simulink model "mg327337"  (Simulink 6.5)
settings: Solver=FixedStepDiscrete  StartTime=0.0  StopTime=20  FixedStep=1  RelTol=1e-3
libraries: simulink x6
CloseFcn:
  | rtwprivate ssgensfun ModelCloseRequest mg327337
settings Model: Creator=mshakeri  LastModifiedBy=mshakeri  ExtModeAutoUpdateStatusClock=off
settings OptimizationCC: InlineParams=on
settings DebuggingCC: SignalResolutionControl=UseLocalSettings  StrictBusMsg=ErrorLevel1

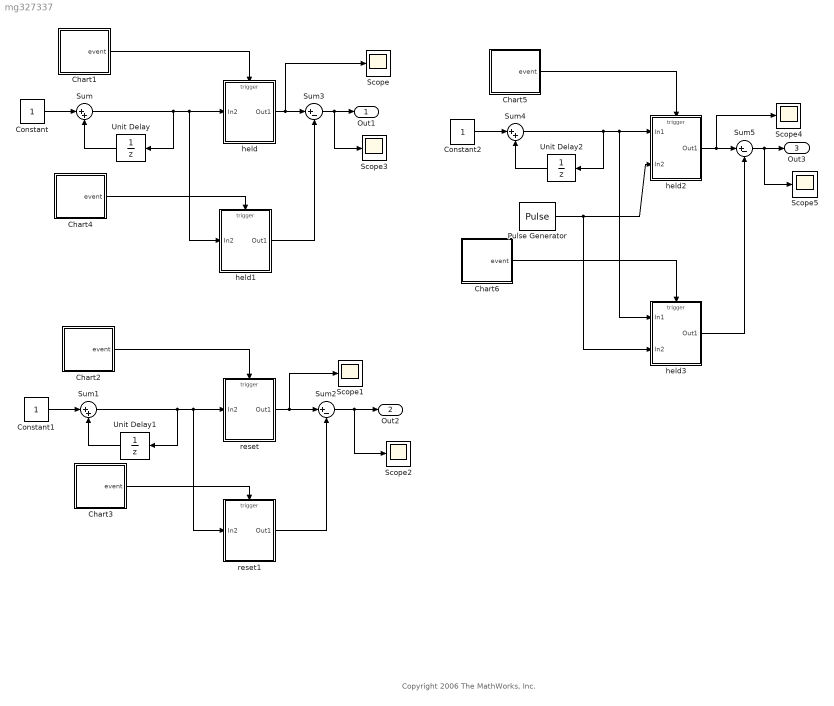
== system mg327337 ==
  note: Copyright 2006 The MathWorks, Inc.
  Chart1 : Stateflow chart  TreatAsAtomicUnit=on  SystemSampleTime=1
  Chart2 : Stateflow chart  TreatAsAtomicUnit=on  SystemSampleTime=1
  Chart3 : Stateflow chart  TreatAsAtomicUnit=on  SystemSampleTime=1
  Chart4 : Stateflow chart  TreatAsAtomicUnit=on  SystemSampleTime=1
  Chart5 : Stateflow chart  TreatAsAtomicUnit=on  SystemSampleTime=1
  Chart6 : Stateflow chart  TreatAsAtomicUnit=on  SystemSampleTime=1
  Constant : Constant
  Constant1 : Constant
  Constant2 : Constant
  Pulse Generator : DiscretePulseGenerator  PulseType=Time based  PulseWidth=50
  Scope{,1..5} (6 alike) : Scope
      Scope2 settings: SaveName=ScopeData2
      Scope3 settings: SaveName=ScopeData3
      Scope4 settings: SaveName=ScopeData4
      Scope5 settings: SaveName=ScopeData5
  Sum : Sum  Inputs=|++
  Sum1 : Sum  Inputs=|++
  Sum2 : Sum  Inputs=|+-
  Sum3 : Sum  Inputs=|+-
  Sum4 : Sum  Inputs=|++
  Sum5 : Sum  Inputs=|+-
  Unit Delay : UnitDelay  Orientation=left
  Unit Delay1 : UnitDelay  Orientation=left
  Unit Delay2 : UnitDelay  Orientation=left
  held : Subsystem  TreatAsAtomicUnit=on
      settings: RTWSystemCode=Inline
  held1 : Subsystem  TreatAsAtomicUnit=on
      settings: RTWSystemCode=Inline
  held2 : Subsystem  TreatAsAtomicUnit=on
      settings: RTWSystemCode=Inline
  held3 : Subsystem  TreatAsAtomicUnit=on
      settings: RTWSystemCode=Inline
  reset : Subsystem  TreatAsAtomicUnit=on
      settings: RTWSystemCode=Inline
  reset1 : Subsystem  TreatAsAtomicUnit=on
      settings: RTWSystemCode=Inline
  Out1 : Outport  InitialOutput=10
  Out2 : Outport  Port=2  InitialOutput=10
  Out3 : Outport  Port=3  InitialOutput=10
  wires:
  Constant/1 -> Sum/1
  Unit Delay/1 -> Sum/2
  Sum/1 -> Unit Delay/1, held/1(In2), held1/1(In2)
  Chart1/1(event) -> held/Trigger
  held/1(Out1) -> Scope/1, Sum3/1
  Constant1/1 -> Sum1/1
  Unit Delay1/1 -> Sum1/2
  Sum1/1 -> Unit Delay1/1, reset/1(In2), reset1/1(In2)
  Chart2/1(event) -> reset/Trigger
  reset/1(Out1) -> Scope1/1, Sum2/1
  Chart3/1(event) -> reset1/Trigger
  reset1/1(Out1) -> Sum2/2
  Sum2/1 -> Out2/1, Scope2/1
  Chart4/1(event) -> held1/Trigger
  held1/1(Out1) -> Sum3/2
  Sum3/1 -> Out1/1, Scope3/1
  Constant2/1 -> Sum4/1
  Unit Delay2/1 -> Sum4/2
  Sum4/1 -> held2/1(In1), held3/1(In1), Unit Delay2/1
  Chart5/1(event) -> held2/Trigger
  Chart6/1(event) -> held3/Trigger
  held3/1(Out1) -> Sum5/2
  Sum5/1 -> Scope5/1, Out3/1
  Pulse Generator/1 -> held2/2(In2), held3/2(In2)
  held2/1(Out1) -> Sum5/1, Scope4/1

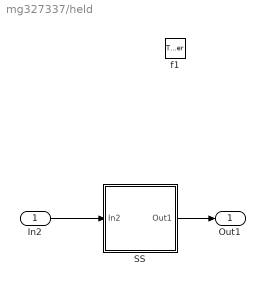
== system mg327337/held ==
  In2 : Inport
  f1 : TriggerPort  TriggerType=function-call
  SS : Subsystem  TreatAsAtomicUnit=on
  Out1 : Outport
  wires:
  In2/1 -> SS/1(In2)
  SS/1(Out1) -> Out1/1

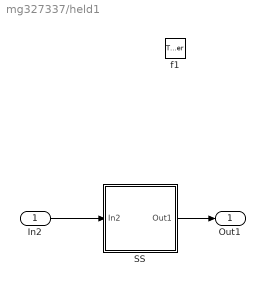
== system mg327337/held1 ==
  In2 : Inport
  f1 : TriggerPort  TriggerType=function-call
  SS : Subsystem  TreatAsAtomicUnit=on
  Out1 : Outport
  wires:
  SS/1(Out1) -> Out1/1
  In2/1 -> SS/1(In2)

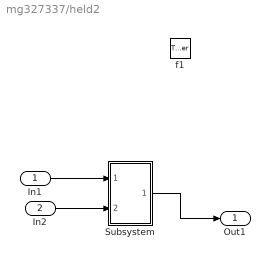
== system mg327337/held2 ==
  In1 : Inport
  In2 : Inport  Port=2
  f1 : TriggerPort  TriggerType=function-call
  Subsystem : Subsystem  TreatAsAtomicUnit=on
  Out1 : Outport
  wires:
  Subsystem/1(Out1) -> Out1/1
  In2/1 -> Subsystem/2(In2)
  In1/1 -> Subsystem/1(In1)

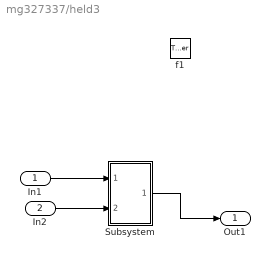
== system mg327337/held3 ==
  In1 : Inport
  In2 : Inport  Port=2
  f1 : TriggerPort  TriggerType=function-call
  Subsystem : Subsystem  TreatAsAtomicUnit=on
  Out1 : Outport
  wires:
  In1/1 -> Subsystem/1(In1)
  In2/1 -> Subsystem/2(In2)
  Subsystem/1(Out1) -> Out1/1

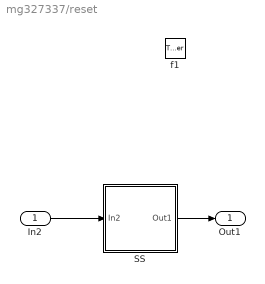
== system mg327337/reset ==
  In2 : Inport
  f1 : TriggerPort  TriggerType=function-call  StatesWhenEnabling=reset
  SS : Subsystem  TreatAsAtomicUnit=on
  Out1 : Outport
  wires:
  SS/1(Out1) -> Out1/1
  In2/1 -> SS/1(In2)

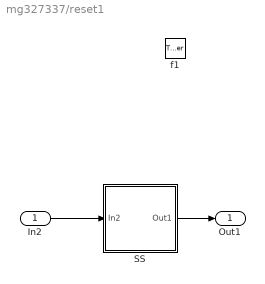
== system mg327337/reset1 ==
  In2 : Inport
  f1 : TriggerPort  TriggerType=function-call  StatesWhenEnabling=reset
  SS : Subsystem  TreatAsAtomicUnit=on
  Out1 : Outport
  wires:
  In2/1 -> SS/1(In2)
  SS/1(Out1) -> Out1/1

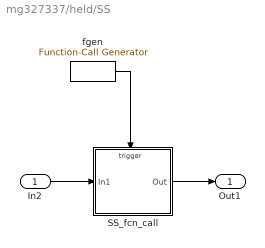
== system mg327337/held/SS ==
  In2 : Inport
  SS_fcn_call : Subsystem  TreatAsAtomicUnit=on  CheckFcnCallInpInsideContextMsg=on  RTWFcnName=foo  RTWFileName=foo
  fgen : simulink/Ports & Subsystems/Function-Call Generator  sample_time=-1  numberOfIterations=1
  Out1 : Outport
  wires:
  fgen/1 -> SS_fcn_call/Trigger
  SS_fcn_call/1(Out) -> Out1/1
  In2/1 -> SS_fcn_call/1(In1)

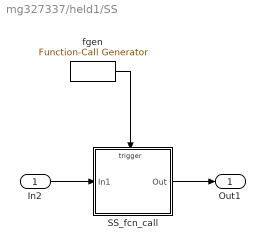
== system mg327337/held1/SS ==
  In2 : Inport
  SS_fcn_call : Subsystem  TreatAsAtomicUnit=on  CheckFcnCallInpInsideContextMsg=on  RTWFcnName=foo  RTWFileName=foo
  fgen : simulink/Ports & Subsystems/Function-Call Generator  sample_time=-1  numberOfIterations=1
  Out1 : Outport
  wires:
  In2/1 -> SS_fcn_call/1(In1)
  SS_fcn_call/1(Out) -> Out1/1
  fgen/1 -> SS_fcn_call/Trigger

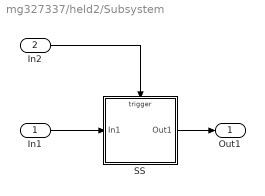
== system mg327337/held2/Subsystem ==
  In1 : Inport
  In2 : Inport  Port=2
  SS : Subsystem  TreatAsAtomicUnit=on
  Out1 : Outport
  wires:
  SS/1(Out1) -> Out1/1
  In1/1 -> SS/1(In1)
  In2/1 -> SS/Trigger

== system mg327337/held3/Subsystem ==
  In1 : Inport
  In2 : Inport  Port=2
  SS : Subsystem  TreatAsAtomicUnit=on
  Out1 : Outport
  wires:
  In2/1 -> SS/Trigger
  In1/1 -> SS/1(In1)
  SS/1(Out1) -> Out1/1

== system mg327337/reset/SS ==
  In2 : Inport
  SS_fcn_call : Subsystem  TreatAsAtomicUnit=on  CheckFcnCallInpInsideContextMsg=on  RTWFcnName=foo  RTWFileName=foo
  fgen : simulink/Ports & Subsystems/Function-Call Generator  sample_time=-1  numberOfIterations=1
  Out1 : Outport
  wires:
  In2/1 -> SS_fcn_call/1(In1)
  SS_fcn_call/1(Out) -> Out1/1
  fgen/1 -> SS_fcn_call/Trigger

== system mg327337/reset1/SS ==
  In2 : Inport
  SS_fcn_call : Subsystem  TreatAsAtomicUnit=on  CheckFcnCallInpInsideContextMsg=on  RTWFcnName=foo  RTWFileName=foo
  fgen : simulink/Ports & Subsystems/Function-Call Generator  sample_time=-1  numberOfIterations=1
  Out1 : Outport
  wires:
  fgen/1 -> SS_fcn_call/Trigger
  SS_fcn_call/1(Out) -> Out1/1
  In2/1 -> SS_fcn_call/1(In1)

== system mg327337/held/SS/SS_fcn_call ==
  In1 : Inport
  f2 : TriggerPort  TriggerType=function-call
  Unit Delay1 : UnitDelay  SampleTime=-1
  Out : Outport  InitialOutput=0
  wires:
  In1/1 -> Unit Delay1/1
  Unit Delay1/1 -> Out/1

== system mg327337/held1/SS/SS_fcn_call ==
  In1 : Inport
  f2 : TriggerPort  TriggerType=function-call
  Unit Delay1 : UnitDelay  SampleTime=-1
  Out : Outport  InitialOutput=0
  wires:
  Unit Delay1/1 -> Out/1
  In1/1 -> Unit Delay1/1

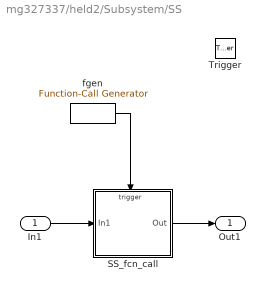
== system mg327337/held2/Subsystem/SS ==
  In1 : Inport
  Trigger : TriggerPort
  SS_fcn_call : Subsystem  TreatAsAtomicUnit=on  CheckFcnCallInpInsideContextMsg=on  RTWFcnName=foo  RTWFileName=foo
  fgen : simulink/Ports & Subsystems/Function-Call Generator  sample_time=-1  numberOfIterations=1
  Out1 : Outport
  wires:
  In1/1 -> SS_fcn_call/1(In1)
  SS_fcn_call/1(Out) -> Out1/1
  fgen/1 -> SS_fcn_call/Trigger

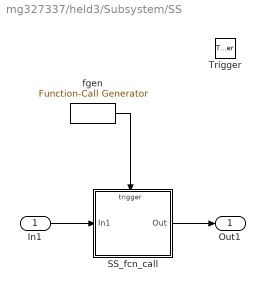
== system mg327337/held3/Subsystem/SS ==
  In1 : Inport
  Trigger : TriggerPort
  SS_fcn_call : Subsystem  TreatAsAtomicUnit=on  CheckFcnCallInpInsideContextMsg=on  RTWFcnName=foo  RTWFileName=foo
  fgen : simulink/Ports & Subsystems/Function-Call Generator  sample_time=-1  numberOfIterations=1
  Out1 : Outport
  wires:
  fgen/1 -> SS_fcn_call/Trigger
  SS_fcn_call/1(Out) -> Out1/1
  In1/1 -> SS_fcn_call/1(In1)

== system mg327337/reset/SS/SS_fcn_call ==
  In1 : Inport
  f2 : TriggerPort  TriggerType=function-call
  Unit Delay1 : UnitDelay  SampleTime=-1
  Out : Outport  InitialOutput=0
  wires:
  Unit Delay1/1 -> Out/1
  In1/1 -> Unit Delay1/1

== system mg327337/reset1/SS/SS_fcn_call ==
  In1 : Inport
  f2 : TriggerPort  TriggerType=function-call
  Unit Delay1 : UnitDelay  SampleTime=-1
  Out : Outport  InitialOutput=0
  wires:
  In1/1 -> Unit Delay1/1
  Unit Delay1/1 -> Out/1

== system mg327337/held2/Subsystem/SS/SS_fcn_call ==
  In1 : Inport
  f2 : TriggerPort  TriggerType=function-call
  Unit Delay1 : UnitDelay  SampleTime=-1
  Out : Outport  InitialOutput=0
  wires:
  In1/1 -> Unit Delay1/1
  Unit Delay1/1 -> Out/1

== system mg327337/held3/Subsystem/SS/SS_fcn_call ==
  In1 : Inport
  f2 : TriggerPort  TriggerType=function-call
  Unit Delay1 : UnitDelay  SampleTime=-1
  Out : Outport  InitialOutput=0
  wires:
  Unit Delay1/1 -> Out/1
  In1/1 -> Unit Delay1/1

== stateflow chart Chart2 ==
  state a
    bind: event;
    en: event;
    du: event;
  state b
  a -> b : after(5,tick)
  b -> a : after(5,tick)
  (default) -> a
  events: event output FUNCTION_CALL_EVENT

== stateflow chart Chart1 ==
  state a
    bind: event;
    en: event;
    du: event;
  state b
  a -> b : after(5,tick)
  b -> a : after(5,tick)
  (default) -> a
  events: event output FUNCTION_CALL_EVENT

== stateflow chart Chart3 ==
  state a
    bind: event;
    en: event;
    du: event;
  state b
  a -> b : after(5,tick)
  b -> a : after(5,tick)
  (default) -> a
  events: event output FUNCTION_CALL_EVENT

== stateflow chart Chart4 ==
  state a
    bind: event;
    en: event;
    du: event;
  state b
  a -> b : after(5,tick)
  b -> a : after(5,tick)
  (default) -> a
  events: event output FUNCTION_CALL_EVENT

== stateflow chart Chart5 ==
  state a
    bind: event;
    en: event;
    du: event;
  state b
  a -> b : after(5,tick)
  b -> a : after(5,tick)
  (default) -> a
  events: event output FUNCTION_CALL_EVENT

== stateflow chart Chart6 ==
  state a
    bind: event;
    en: event;
    du: event;
  state b
  a -> b : after(5,tick)
  b -> a : after(5,tick)
  (default) -> a
  events: event output FUNCTION_CALL_EVENT
